simulink model "nn_12B_with_contracts_SLDV"  (R2019b)
settings: Solver=FixedStepDiscrete  StartTime=0  StopTime=100  FixedStep=1  RelTol=1e-3  EnableMultiTasking=on
model workspace (MAT data in the model file):
  ContractValidatorBlocksMap : containers.Map (value not decoded)
undefined symbols (not defined in the file): b1, b2, b3, meaninp, meanout, oostdinp, stdevout, w1, w2, w3, xinmax, xinmin
libraries: sldvlib x5, cocosimLibs x4
(part 2 of 2)

== system nn_12B_with_contracts_SLDV/nn_2x10x10x1/Neuron Layer 1/Neuron 3/If Action Subsystem1 ==
  In1 : Inport
  Action Port : ActionPort  ActionPortLabel=elseif(u1 < 0)
  Product1 : Product  RndMeth=Zero
  Sum3 : Sum  Inputs=|++
  bias4 : Constant  Value=2
  Out1 : Outport  VectorParamsAs1DForOutWhenUnconnected=off
  wires:
  In1/1 -> Product1/1, Sum3/1
  bias4/1 -> Sum3/2
  Sum3/1 -> Product1/2
  Product1/1 -> Out1/1

== system nn_12B_with_contracts_SLDV/nn_2x10x10x1/Neuron Layer 1/Neuron 3/If Action Subsystem2 ==
  In1 : Inport
  Action Port : ActionPort  ActionPortLabel=elseif( u1<0.995)
  Product1 : Product  RndMeth=Zero
  Sum3 : Sum  Inputs=|-+
  bias4 : Constant  Value=2
  Out1 : Outport  VectorParamsAs1DForOutWhenUnconnected=off
  wires:
  Product1/1 -> Out1/1
  Sum3/1 -> Product1/2
  bias4/1 -> Sum3/2
  In1/1 -> Sum3/1, Product1/1

== system nn_12B_with_contracts_SLDV/nn_2x10x10x1/Neuron Layer 1/Neuron 3/If Action Subsystem3 ==
  In1 : Inport
  Action Port : ActionPort  ActionPortLabel=else
  Sum : Sum  Inputs=|++
  bias1 : Constant  Value=0.990025
  weight1 : Gain  Gain=0.01
  Out1 : Outport  VectorParamsAs1DForOutWhenUnconnected=off
  wires:
  bias1/1 -> Sum/2
  weight1/1 -> Sum/1
  In1/1 -> weight1/1
  Sum/1 -> Out1/1

== system nn_12B_with_contracts_SLDV/nn_2x10x10x1/Neuron Layer 1/Neuron 4/If Action Subsystem ==
  In1 : Inport
  Action Port : ActionPort  ActionPortLabel=if(u1 < -0.995)
  Sum : Sum  Inputs=|+-
  bias1 : Constant  Value=0.990025
  weight1 : Gain  Gain=0.01
  Out1 : Outport  VectorParamsAs1DForOutWhenUnconnected=off
  wires:
  bias1/1 -> Sum/2
  weight1/1 -> Sum/1
  In1/1 -> weight1/1
  Sum/1 -> Out1/1

== system nn_12B_with_contracts_SLDV/nn_2x10x10x1/Neuron Layer 1/Neuron 4/If Action Subsystem1 ==
  In1 : Inport
  Action Port : ActionPort  ActionPortLabel=elseif(u1 < 0)
  Product1 : Product  RndMeth=Zero
  Sum3 : Sum  Inputs=|++
  bias4 : Constant  Value=2
  Out1 : Outport  VectorParamsAs1DForOutWhenUnconnected=off
  wires:
  In1/1 -> Product1/1, Sum3/1
  bias4/1 -> Sum3/2
  Sum3/1 -> Product1/2
  Product1/1 -> Out1/1

== system nn_12B_with_contracts_SLDV/nn_2x10x10x1/Neuron Layer 1/Neuron 4/If Action Subsystem2 ==
  In1 : Inport
  Action Port : ActionPort  ActionPortLabel=elseif( u1<0.995)
  Product1 : Product  RndMeth=Zero
  Sum3 : Sum  Inputs=|-+
  bias4 : Constant  Value=2
  Out1 : Outport  VectorParamsAs1DForOutWhenUnconnected=off
  wires:
  Product1/1 -> Out1/1
  Sum3/1 -> Product1/2
  bias4/1 -> Sum3/2
  In1/1 -> Sum3/1, Product1/1

== system nn_12B_with_contracts_SLDV/nn_2x10x10x1/Neuron Layer 1/Neuron 4/If Action Subsystem3 ==
  In1 : Inport
  Action Port : ActionPort  ActionPortLabel=else
  Sum : Sum  Inputs=|++
  bias1 : Constant  Value=0.990025
  weight1 : Gain  Gain=0.01
  Out1 : Outport  VectorParamsAs1DForOutWhenUnconnected=off
  wires:
  bias1/1 -> Sum/2
  weight1/1 -> Sum/1
  In1/1 -> weight1/1
  Sum/1 -> Out1/1

== system nn_12B_with_contracts_SLDV/nn_2x10x10x1/Neuron Layer 1/Neuron 5/If Action Subsystem ==
  In1 : Inport
  Action Port : ActionPort  ActionPortLabel=if(u1 < -0.995)
  Sum : Sum  Inputs=|+-
  bias1 : Constant  Value=0.990025
  weight1 : Gain  Gain=0.01
  Out1 : Outport  VectorParamsAs1DForOutWhenUnconnected=off
  wires:
  bias1/1 -> Sum/2
  weight1/1 -> Sum/1
  In1/1 -> weight1/1
  Sum/1 -> Out1/1

== system nn_12B_with_contracts_SLDV/nn_2x10x10x1/Neuron Layer 1/Neuron 5/If Action Subsystem1 ==
  In1 : Inport
  Action Port : ActionPort  ActionPortLabel=elseif(u1 < 0)
  Product1 : Product  RndMeth=Zero
  Sum3 : Sum  Inputs=|++
  bias4 : Constant  Value=2
  Out1 : Outport  VectorParamsAs1DForOutWhenUnconnected=off
  wires:
  In1/1 -> Product1/1, Sum3/1
  bias4/1 -> Sum3/2
  Sum3/1 -> Product1/2
  Product1/1 -> Out1/1

== system nn_12B_with_contracts_SLDV/nn_2x10x10x1/Neuron Layer 1/Neuron 5/If Action Subsystem2 ==
  In1 : Inport
  Action Port : ActionPort  ActionPortLabel=elseif( u1<0.995)
  Product1 : Product  RndMeth=Zero
  Sum3 : Sum  Inputs=|-+
  bias4 : Constant  Value=2
  Out1 : Outport  VectorParamsAs1DForOutWhenUnconnected=off
  wires:
  Product1/1 -> Out1/1
  Sum3/1 -> Product1/2
  bias4/1 -> Sum3/2
  In1/1 -> Sum3/1, Product1/1

== system nn_12B_with_contracts_SLDV/nn_2x10x10x1/Neuron Layer 1/Neuron 5/If Action Subsystem3 ==
  In1 : Inport
  Action Port : ActionPort  ActionPortLabel=else
  Sum : Sum  Inputs=|++
  bias1 : Constant  Value=0.990025
  weight1 : Gain  Gain=0.01
  Out1 : Outport  VectorParamsAs1DForOutWhenUnconnected=off
  wires:
  bias1/1 -> Sum/2
  weight1/1 -> Sum/1
  In1/1 -> weight1/1
  Sum/1 -> Out1/1

== system nn_12B_with_contracts_SLDV/nn_2x10x10x1/Neuron Layer 1/Neuron 6/If Action Subsystem ==
  In1 : Inport
  Action Port : ActionPort  ActionPortLabel=if(u1 < -0.995)
  Sum : Sum  Inputs=|+-
  bias1 : Constant  Value=0.990025
  weight1 : Gain  Gain=0.01
  Out1 : Outport  VectorParamsAs1DForOutWhenUnconnected=off
  wires:
  Sum/1 -> Out1/1
  In1/1 -> weight1/1
  weight1/1 -> Sum/1
  bias1/1 -> Sum/2

== system nn_12B_with_contracts_SLDV/nn_2x10x10x1/Neuron Layer 1/Neuron 6/If Action Subsystem1 ==
  In1 : Inport
  Action Port : ActionPort  ActionPortLabel=elseif(u1 < 0)
  Product1 : Product  RndMeth=Zero
  Sum3 : Sum  Inputs=|++
  bias4 : Constant  Value=2
  Out1 : Outport  VectorParamsAs1DForOutWhenUnconnected=off
  wires:
  Product1/1 -> Out1/1
  Sum3/1 -> Product1/2
  bias4/1 -> Sum3/2
  In1/1 -> Sum3/1, Product1/1

== system nn_12B_with_contracts_SLDV/nn_2x10x10x1/Neuron Layer 1/Neuron 6/If Action Subsystem2 ==
  In1 : Inport
  Action Port : ActionPort  ActionPortLabel=elseif( u1<0.995)
  Product1 : Product  RndMeth=Zero
  Sum3 : Sum  Inputs=|-+
  bias4 : Constant  Value=2
  Out1 : Outport  VectorParamsAs1DForOutWhenUnconnected=off
  wires:
  In1/1 -> Product1/1, Sum3/1
  bias4/1 -> Sum3/2
  Sum3/1 -> Product1/2
  Product1/1 -> Out1/1

== system nn_12B_with_contracts_SLDV/nn_2x10x10x1/Neuron Layer 1/Neuron 6/If Action Subsystem3 ==
  In1 : Inport
  Action Port : ActionPort  ActionPortLabel=else
  Sum : Sum  Inputs=|++
  bias1 : Constant  Value=0.990025
  weight1 : Gain  Gain=0.01
  Out1 : Outport  VectorParamsAs1DForOutWhenUnconnected=off
  wires:
  Sum/1 -> Out1/1
  In1/1 -> weight1/1
  weight1/1 -> Sum/1
  bias1/1 -> Sum/2

== system nn_12B_with_contracts_SLDV/nn_2x10x10x1/Neuron Layer 1/Neuron 7/If Action Subsystem ==
  In1 : Inport
  Action Port : ActionPort  ActionPortLabel=if(u1 < -0.995)
  Sum : Sum  Inputs=|+-
  bias1 : Constant  Value=0.990025
  weight1 : Gain  Gain=0.01
  Out1 : Outport  VectorParamsAs1DForOutWhenUnconnected=off
  wires:
  bias1/1 -> Sum/2
  weight1/1 -> Sum/1
  In1/1 -> weight1/1
  Sum/1 -> Out1/1

== system nn_12B_with_contracts_SLDV/nn_2x10x10x1/Neuron Layer 1/Neuron 7/If Action Subsystem1 ==
  In1 : Inport
  Action Port : ActionPort  ActionPortLabel=elseif(u1 < 0)
  Product1 : Product  RndMeth=Zero
  Sum3 : Sum  Inputs=|++
  bias4 : Constant  Value=2
  Out1 : Outport  VectorParamsAs1DForOutWhenUnconnected=off
  wires:
  In1/1 -> Product1/1, Sum3/1
  bias4/1 -> Sum3/2
  Sum3/1 -> Product1/2
  Product1/1 -> Out1/1

== system nn_12B_with_contracts_SLDV/nn_2x10x10x1/Neuron Layer 1/Neuron 7/If Action Subsystem2 ==
  In1 : Inport
  Action Port : ActionPort  ActionPortLabel=elseif( u1<0.995)
  Product1 : Product  RndMeth=Zero
  Sum3 : Sum  Inputs=|-+
  bias4 : Constant  Value=2
  Out1 : Outport  VectorParamsAs1DForOutWhenUnconnected=off
  wires:
  Product1/1 -> Out1/1
  Sum3/1 -> Product1/2
  bias4/1 -> Sum3/2
  In1/1 -> Sum3/1, Product1/1

== system nn_12B_with_contracts_SLDV/nn_2x10x10x1/Neuron Layer 1/Neuron 7/If Action Subsystem3 ==
  In1 : Inport
  Action Port : ActionPort  ActionPortLabel=else
  Sum : Sum  Inputs=|++
  bias1 : Constant  Value=0.990025
  weight1 : Gain  Gain=0.01
  Out1 : Outport  VectorParamsAs1DForOutWhenUnconnected=off
  wires:
  bias1/1 -> Sum/2
  weight1/1 -> Sum/1
  In1/1 -> weight1/1
  Sum/1 -> Out1/1

== system nn_12B_with_contracts_SLDV/nn_2x10x10x1/Neuron Layer 1/Neuron 8/If Action Subsystem ==
  In1 : Inport
  Action Port : ActionPort  ActionPortLabel=if(u1 < -0.995)
  Sum : Sum  Inputs=|+-
  bias1 : Constant  Value=0.990025
  weight1 : Gain  Gain=0.01
  Out1 : Outport  VectorParamsAs1DForOutWhenUnconnected=off
  wires:
  bias1/1 -> Sum/2
  weight1/1 -> Sum/1
  In1/1 -> weight1/1
  Sum/1 -> Out1/1

== system nn_12B_with_contracts_SLDV/nn_2x10x10x1/Neuron Layer 1/Neuron 8/If Action Subsystem1 ==
  In1 : Inport
  Action Port : ActionPort  ActionPortLabel=elseif(u1 < 0)
  Product1 : Product  RndMeth=Zero
  Sum3 : Sum  Inputs=|++
  bias4 : Constant  Value=2
  Out1 : Outport  VectorParamsAs1DForOutWhenUnconnected=off
  wires:
  In1/1 -> Product1/1, Sum3/1
  bias4/1 -> Sum3/2
  Sum3/1 -> Product1/2
  Product1/1 -> Out1/1

== system nn_12B_with_contracts_SLDV/nn_2x10x10x1/Neuron Layer 1/Neuron 8/If Action Subsystem2 ==
  In1 : Inport
  Action Port : ActionPort  ActionPortLabel=elseif( u1<0.995)
  Product1 : Product  RndMeth=Zero
  Sum3 : Sum  Inputs=|-+
  bias4 : Constant  Value=2
  Out1 : Outport  VectorParamsAs1DForOutWhenUnconnected=off
  wires:
  Product1/1 -> Out1/1
  Sum3/1 -> Product1/2
  bias4/1 -> Sum3/2
  In1/1 -> Sum3/1, Product1/1

== system nn_12B_with_contracts_SLDV/nn_2x10x10x1/Neuron Layer 1/Neuron 8/If Action Subsystem3 ==
  In1 : Inport
  Action Port : ActionPort  ActionPortLabel=else
  Sum : Sum  Inputs=|++
  bias1 : Constant  Value=0.990025
  weight1 : Gain  Gain=0.01
  Out1 : Outport  VectorParamsAs1DForOutWhenUnconnected=off
  wires:
  bias1/1 -> Sum/2
  weight1/1 -> Sum/1
  In1/1 -> weight1/1
  Sum/1 -> Out1/1

== system nn_12B_with_contracts_SLDV/nn_2x10x10x1/Neuron Layer 1/Neuron 9/If Action Subsystem ==
  In1 : Inport
  Action Port : ActionPort  ActionPortLabel=if(u1 < -0.995)
  Sum : Sum  Inputs=|+-
  bias1 : Constant  Value=0.990025
  weight1 : Gain  Gain=0.01
  Out1 : Outport  VectorParamsAs1DForOutWhenUnconnected=off
  wires:
  bias1/1 -> Sum/2
  weight1/1 -> Sum/1
  In1/1 -> weight1/1
  Sum/1 -> Out1/1

== system nn_12B_with_contracts_SLDV/nn_2x10x10x1/Neuron Layer 1/Neuron 9/If Action Subsystem1 ==
  In1 : Inport
  Action Port : ActionPort  ActionPortLabel=elseif(u1 < 0)
  Product1 : Product  RndMeth=Zero
  Sum3 : Sum  Inputs=|++
  bias4 : Constant  Value=2
  Out1 : Outport  VectorParamsAs1DForOutWhenUnconnected=off
  wires:
  In1/1 -> Product1/1, Sum3/1
  bias4/1 -> Sum3/2
  Sum3/1 -> Product1/2
  Product1/1 -> Out1/1

== system nn_12B_with_contracts_SLDV/nn_2x10x10x1/Neuron Layer 1/Neuron 9/If Action Subsystem2 ==
  In1 : Inport
  Action Port : ActionPort  ActionPortLabel=elseif( u1<0.995)
  Product1 : Product  RndMeth=Zero
  Sum3 : Sum  Inputs=|-+
  bias4 : Constant  Value=2
  Out1 : Outport  VectorParamsAs1DForOutWhenUnconnected=off
  wires:
  Product1/1 -> Out1/1
  Sum3/1 -> Product1/2
  bias4/1 -> Sum3/2
  In1/1 -> Sum3/1, Product1/1

== system nn_12B_with_contracts_SLDV/nn_2x10x10x1/Neuron Layer 1/Neuron 9/If Action Subsystem3 ==
  In1 : Inport
  Action Port : ActionPort  ActionPortLabel=else
  Sum : Sum  Inputs=|++
  bias1 : Constant  Value=0.990025
  weight1 : Gain  Gain=0.01
  Out1 : Outport  VectorParamsAs1DForOutWhenUnconnected=off
  wires:
  bias1/1 -> Sum/2
  weight1/1 -> Sum/1
  In1/1 -> weight1/1
  Sum/1 -> Out1/1

== system nn_12B_with_contracts_SLDV/nn_2x10x10x1/Neuron Layer 2/Neuron 1/If Action Subsystem ==
  In1 : Inport
  Action Port : ActionPort  ActionPortLabel=if(u1 < -0.995)
  Sum : Sum  Inputs=|+-
  bias1 : Constant  Value=0.990025
  weight1 : Gain  Gain=0.01
  Out1 : Outport  VectorParamsAs1DForOutWhenUnconnected=off
  wires:
  bias1/1 -> Sum/2
  weight1/1 -> Sum/1
  In1/1 -> weight1/1
  Sum/1 -> Out1/1

== system nn_12B_with_contracts_SLDV/nn_2x10x10x1/Neuron Layer 2/Neuron 1/If Action Subsystem1 ==
  In1 : Inport
  Action Port : ActionPort  ActionPortLabel=elseif(u1 < 0)
  Product1 : Product  RndMeth=Zero
  Sum3 : Sum  Inputs=|++
  bias4 : Constant  Value=2
  Out1 : Outport  VectorParamsAs1DForOutWhenUnconnected=off
  wires:
  In1/1 -> Product1/1, Sum3/1
  bias4/1 -> Sum3/2
  Sum3/1 -> Product1/2
  Product1/1 -> Out1/1

== system nn_12B_with_contracts_SLDV/nn_2x10x10x1/Neuron Layer 2/Neuron 1/If Action Subsystem2 ==
  In1 : Inport
  Action Port : ActionPort  ActionPortLabel=elseif( u1<0.995)
  Product1 : Product  RndMeth=Zero
  Sum3 : Sum  Inputs=|-+
  bias4 : Constant  Value=2
  Out1 : Outport  VectorParamsAs1DForOutWhenUnconnected=off
  wires:
  Product1/1 -> Out1/1
  Sum3/1 -> Product1/2
  bias4/1 -> Sum3/2
  In1/1 -> Sum3/1, Product1/1

== system nn_12B_with_contracts_SLDV/nn_2x10x10x1/Neuron Layer 2/Neuron 1/If Action Subsystem3 ==
  In1 : Inport
  Action Port : ActionPort  ActionPortLabel=else
  Sum : Sum  Inputs=|++
  bias1 : Constant  Value=0.990025
  weight1 : Gain  Gain=0.01
  Out1 : Outport  VectorParamsAs1DForOutWhenUnconnected=off
  wires:
  bias1/1 -> Sum/2
  weight1/1 -> Sum/1
  In1/1 -> weight1/1
  Sum/1 -> Out1/1

== system nn_12B_with_contracts_SLDV/nn_2x10x10x1/Neuron Layer 2/Neuron 10/If Action Subsystem ==
  In1 : Inport
  Action Port : ActionPort  ActionPortLabel=if(u1 < -0.995)
  Sum : Sum  Inputs=|+-
  bias1 : Constant  Value=0.990025
  weight1 : Gain  Gain=0.01
  Out1 : Outport  VectorParamsAs1DForOutWhenUnconnected=off
  wires:
  Sum/1 -> Out1/1
  In1/1 -> weight1/1
  weight1/1 -> Sum/1
  bias1/1 -> Sum/2

== system nn_12B_with_contracts_SLDV/nn_2x10x10x1/Neuron Layer 2/Neuron 10/If Action Subsystem1 ==
  In1 : Inport
  Action Port : ActionPort  ActionPortLabel=elseif(u1 < 0)
  Product1 : Product  RndMeth=Zero
  Sum3 : Sum  Inputs=|++
  bias4 : Constant  Value=2
  Out1 : Outport  VectorParamsAs1DForOutWhenUnconnected=off
  wires:
  Product1/1 -> Out1/1
  Sum3/1 -> Product1/2
  bias4/1 -> Sum3/2
  In1/1 -> Sum3/1, Product1/1

== system nn_12B_with_contracts_SLDV/nn_2x10x10x1/Neuron Layer 2/Neuron 10/If Action Subsystem2 ==
  In1 : Inport
  Action Port : ActionPort  ActionPortLabel=elseif( u1<0.995)
  Product1 : Product  RndMeth=Zero
  Sum3 : Sum  Inputs=|-+
  bias4 : Constant  Value=2
  Out1 : Outport  VectorParamsAs1DForOutWhenUnconnected=off
  wires:
  In1/1 -> Product1/1, Sum3/1
  bias4/1 -> Sum3/2
  Sum3/1 -> Product1/2
  Product1/1 -> Out1/1

== system nn_12B_with_contracts_SLDV/nn_2x10x10x1/Neuron Layer 2/Neuron 10/If Action Subsystem3 ==
  In1 : Inport
  Action Port : ActionPort  ActionPortLabel=else
  Sum : Sum  Inputs=|++
  bias1 : Constant  Value=0.990025
  weight1 : Gain  Gain=0.01
  Out1 : Outport  VectorParamsAs1DForOutWhenUnconnected=off
  wires:
  Sum/1 -> Out1/1
  In1/1 -> weight1/1
  weight1/1 -> Sum/1
  bias1/1 -> Sum/2

== system nn_12B_with_contracts_SLDV/nn_2x10x10x1/Neuron Layer 2/Neuron 2/If Action Subsystem ==
  In1 : Inport
  Action Port : ActionPort  ActionPortLabel=if(u1 < -0.995)
  Sum : Sum  Inputs=|+-
  bias1 : Constant  Value=0.990025
  weight1 : Gain  Gain=0.01
  Out1 : Outport  VectorParamsAs1DForOutWhenUnconnected=off
  wires:
  Sum/1 -> Out1/1
  In1/1 -> weight1/1
  weight1/1 -> Sum/1
  bias1/1 -> Sum/2

== system nn_12B_with_contracts_SLDV/nn_2x10x10x1/Neuron Layer 2/Neuron 2/If Action Subsystem1 ==
  In1 : Inport
  Action Port : ActionPort  ActionPortLabel=elseif(u1 < 0)
  Product1 : Product  RndMeth=Zero
  Sum3 : Sum  Inputs=|++
  bias4 : Constant  Value=2
  Out1 : Outport  VectorParamsAs1DForOutWhenUnconnected=off
  wires:
  Product1/1 -> Out1/1
  Sum3/1 -> Product1/2
  bias4/1 -> Sum3/2
  In1/1 -> Sum3/1, Product1/1

== system nn_12B_with_contracts_SLDV/nn_2x10x10x1/Neuron Layer 2/Neuron 2/If Action Subsystem2 ==
  In1 : Inport
  Action Port : ActionPort  ActionPortLabel=elseif( u1<0.995)
  Product1 : Product  RndMeth=Zero
  Sum3 : Sum  Inputs=|-+
  bias4 : Constant  Value=2
  Out1 : Outport  VectorParamsAs1DForOutWhenUnconnected=off
  wires:
  In1/1 -> Product1/1, Sum3/1
  bias4/1 -> Sum3/2
  Sum3/1 -> Product1/2
  Product1/1 -> Out1/1

== system nn_12B_with_contracts_SLDV/nn_2x10x10x1/Neuron Layer 2/Neuron 2/If Action Subsystem3 ==
  In1 : Inport
  Action Port : ActionPort  ActionPortLabel=else
  Sum : Sum  Inputs=|++
  bias1 : Constant  Value=0.990025
  weight1 : Gain  Gain=0.01
  Out1 : Outport  VectorParamsAs1DForOutWhenUnconnected=off
  wires:
  Sum/1 -> Out1/1
  In1/1 -> weight1/1
  weight1/1 -> Sum/1
  bias1/1 -> Sum/2

== system nn_12B_with_contracts_SLDV/nn_2x10x10x1/Neuron Layer 2/Neuron 3/If Action Subsystem ==
  In1 : Inport
  Action Port : ActionPort  ActionPortLabel=if(u1 < -0.995)
  Sum : Sum  Inputs=|+-
  bias1 : Constant  Value=0.990025
  weight1 : Gain  Gain=0.01
  Out1 : Outport  VectorParamsAs1DForOutWhenUnconnected=off
  wires:
  bias1/1 -> Sum/2
  weight1/1 -> Sum/1
  In1/1 -> weight1/1
  Sum/1 -> Out1/1

== system nn_12B_with_contracts_SLDV/nn_2x10x10x1/Neuron Layer 2/Neuron 3/If Action Subsystem1 ==
  In1 : Inport
  Action Port : ActionPort  ActionPortLabel=elseif(u1 < 0)
  Product1 : Product  RndMeth=Zero
  Sum3 : Sum  Inputs=|++
  bias4 : Constant  Value=2
  Out1 : Outport  VectorParamsAs1DForOutWhenUnconnected=off
  wires:
  In1/1 -> Product1/1, Sum3/1
  bias4/1 -> Sum3/2
  Sum3/1 -> Product1/2
  Product1/1 -> Out1/1

== system nn_12B_with_contracts_SLDV/nn_2x10x10x1/Neuron Layer 2/Neuron 3/If Action Subsystem2 ==
  In1 : Inport
  Action Port : ActionPort  ActionPortLabel=elseif( u1<0.995)
  Product1 : Product  RndMeth=Zero
  Sum3 : Sum  Inputs=|-+
  bias4 : Constant  Value=2
  Out1 : Outport  VectorParamsAs1DForOutWhenUnconnected=off
  wires:
  Product1/1 -> Out1/1
  Sum3/1 -> Product1/2
  bias4/1 -> Sum3/2
  In1/1 -> Sum3/1, Product1/1

== system nn_12B_with_contracts_SLDV/nn_2x10x10x1/Neuron Layer 2/Neuron 3/If Action Subsystem3 ==
  In1 : Inport
  Action Port : ActionPort  ActionPortLabel=else
  Sum : Sum  Inputs=|++
  bias1 : Constant  Value=0.990025
  weight1 : Gain  Gain=0.01
  Out1 : Outport  VectorParamsAs1DForOutWhenUnconnected=off
  wires:
  bias1/1 -> Sum/2
  weight1/1 -> Sum/1
  In1/1 -> weight1/1
  Sum/1 -> Out1/1

== system nn_12B_with_contracts_SLDV/nn_2x10x10x1/Neuron Layer 2/Neuron 4/If Action Subsystem ==
  In1 : Inport
  Action Port : ActionPort  ActionPortLabel=if(u1 < -0.995)
  Sum : Sum  Inputs=|+-
  bias1 : Constant  Value=0.990025
  weight1 : Gain  Gain=0.01
  Out1 : Outport  VectorParamsAs1DForOutWhenUnconnected=off
  wires:
  bias1/1 -> Sum/2
  weight1/1 -> Sum/1
  In1/1 -> weight1/1
  Sum/1 -> Out1/1

== system nn_12B_with_contracts_SLDV/nn_2x10x10x1/Neuron Layer 2/Neuron 4/If Action Subsystem1 ==
  In1 : Inport
  Action Port : ActionPort  ActionPortLabel=elseif(u1 < 0)
  Product1 : Product  RndMeth=Zero
  Sum3 : Sum  Inputs=|++
  bias4 : Constant  Value=2
  Out1 : Outport  VectorParamsAs1DForOutWhenUnconnected=off
  wires:
  In1/1 -> Product1/1, Sum3/1
  bias4/1 -> Sum3/2
  Sum3/1 -> Product1/2
  Product1/1 -> Out1/1

== system nn_12B_with_contracts_SLDV/nn_2x10x10x1/Neuron Layer 2/Neuron 4/If Action Subsystem2 ==
  In1 : Inport
  Action Port : ActionPort  ActionPortLabel=elseif( u1<0.995)
  Product1 : Product  RndMeth=Zero
  Sum3 : Sum  Inputs=|-+
  bias4 : Constant  Value=2
  Out1 : Outport  VectorParamsAs1DForOutWhenUnconnected=off
  wires:
  Product1/1 -> Out1/1
  Sum3/1 -> Product1/2
  bias4/1 -> Sum3/2
  In1/1 -> Sum3/1, Product1/1

== system nn_12B_with_contracts_SLDV/nn_2x10x10x1/Neuron Layer 2/Neuron 4/If Action Subsystem3 ==
  In1 : Inport
  Action Port : ActionPort  ActionPortLabel=else
  Sum : Sum  Inputs=|++
  bias1 : Constant  Value=0.990025
  weight1 : Gain  Gain=0.01
  Out1 : Outport  VectorParamsAs1DForOutWhenUnconnected=off
  wires:
  bias1/1 -> Sum/2
  weight1/1 -> Sum/1
  In1/1 -> weight1/1
  Sum/1 -> Out1/1

== system nn_12B_with_contracts_SLDV/nn_2x10x10x1/Neuron Layer 2/Neuron 5/If Action Subsystem ==
  In1 : Inport
  Action Port : ActionPort  ActionPortLabel=if(u1 < -0.995)
  Sum : Sum  Inputs=|+-
  bias1 : Constant  Value=0.990025
  weight1 : Gain  Gain=0.01
  Out1 : Outport  VectorParamsAs1DForOutWhenUnconnected=off
  wires:
  bias1/1 -> Sum/2
  weight1/1 -> Sum/1
  In1/1 -> weight1/1
  Sum/1 -> Out1/1

== system nn_12B_with_contracts_SLDV/nn_2x10x10x1/Neuron Layer 2/Neuron 5/If Action Subsystem1 ==
  In1 : Inport
  Action Port : ActionPort  ActionPortLabel=elseif(u1 < 0)
  Product1 : Product  RndMeth=Zero
  Sum3 : Sum  Inputs=|++
  bias4 : Constant  Value=2
  Out1 : Outport  VectorParamsAs1DForOutWhenUnconnected=off
  wires:
  In1/1 -> Product1/1, Sum3/1
  bias4/1 -> Sum3/2
  Sum3/1 -> Product1/2
  Product1/1 -> Out1/1

== system nn_12B_with_contracts_SLDV/nn_2x10x10x1/Neuron Layer 2/Neuron 5/If Action Subsystem2 ==
  In1 : Inport
  Action Port : ActionPort  ActionPortLabel=elseif( u1<0.995)
  Product1 : Product  RndMeth=Zero
  Sum3 : Sum  Inputs=|-+
  bias4 : Constant  Value=2
  Out1 : Outport  VectorParamsAs1DForOutWhenUnconnected=off
  wires:
  Product1/1 -> Out1/1
  Sum3/1 -> Product1/2
  bias4/1 -> Sum3/2
  In1/1 -> Sum3/1, Product1/1

== system nn_12B_with_contracts_SLDV/nn_2x10x10x1/Neuron Layer 2/Neuron 5/If Action Subsystem3 ==
  In1 : Inport
  Action Port : ActionPort  ActionPortLabel=else
  Sum : Sum  Inputs=|++
  bias1 : Constant  Value=0.990025
  weight1 : Gain  Gain=0.01
  Out1 : Outport  VectorParamsAs1DForOutWhenUnconnected=off
  wires:
  bias1/1 -> Sum/2
  weight1/1 -> Sum/1
  In1/1 -> weight1/1
  Sum/1 -> Out1/1

== system nn_12B_with_contracts_SLDV/nn_2x10x10x1/Neuron Layer 2/Neuron 6/If Action Subsystem ==
  In1 : Inport
  Action Port : ActionPort  ActionPortLabel=if(u1 < -0.995)
  Sum : Sum  Inputs=|+-
  bias1 : Constant  Value=0.990025
  weight1 : Gain  Gain=0.01
  Out1 : Outport  VectorParamsAs1DForOutWhenUnconnected=off
  wires:
  Sum/1 -> Out1/1
  In1/1 -> weight1/1
  weight1/1 -> Sum/1
  bias1/1 -> Sum/2

== system nn_12B_with_contracts_SLDV/nn_2x10x10x1/Neuron Layer 2/Neuron 6/If Action Subsystem1 ==
  In1 : Inport
  Action Port : ActionPort  ActionPortLabel=elseif(u1 < 0)
  Product1 : Product  RndMeth=Zero
  Sum3 : Sum  Inputs=|++
  bias4 : Constant  Value=2
  Out1 : Outport  VectorParamsAs1DForOutWhenUnconnected=off
  wires:
  Product1/1 -> Out1/1
  Sum3/1 -> Product1/2
  bias4/1 -> Sum3/2
  In1/1 -> Sum3/1, Product1/1

== system nn_12B_with_contracts_SLDV/nn_2x10x10x1/Neuron Layer 2/Neuron 6/If Action Subsystem2 ==
  In1 : Inport
  Action Port : ActionPort  ActionPortLabel=elseif( u1<0.995)
  Product1 : Product  RndMeth=Zero
  Sum3 : Sum  Inputs=|-+
  bias4 : Constant  Value=2
  Out1 : Outport  VectorParamsAs1DForOutWhenUnconnected=off
  wires:
  In1/1 -> Product1/1, Sum3/1
  bias4/1 -> Sum3/2
  Sum3/1 -> Product1/2
  Product1/1 -> Out1/1

== system nn_12B_with_contracts_SLDV/nn_2x10x10x1/Neuron Layer 2/Neuron 6/If Action Subsystem3 ==
  In1 : Inport
  Action Port : ActionPort  ActionPortLabel=else
  Sum : Sum  Inputs=|++
  bias1 : Constant  Value=0.990025
  weight1 : Gain  Gain=0.01
  Out1 : Outport  VectorParamsAs1DForOutWhenUnconnected=off
  wires:
  Sum/1 -> Out1/1
  In1/1 -> weight1/1
  weight1/1 -> Sum/1
  bias1/1 -> Sum/2

== system nn_12B_with_contracts_SLDV/nn_2x10x10x1/Neuron Layer 2/Neuron 7/If Action Subsystem ==
  In1 : Inport
  Action Port : ActionPort  ActionPortLabel=if(u1 < -0.995)
  Sum : Sum  Inputs=|+-
  bias1 : Constant  Value=0.990025
  weight1 : Gain  Gain=0.01
  Out1 : Outport  VectorParamsAs1DForOutWhenUnconnected=off
  wires:
  bias1/1 -> Sum/2
  weight1/1 -> Sum/1
  In1/1 -> weight1/1
  Sum/1 -> Out1/1

== system nn_12B_with_contracts_SLDV/nn_2x10x10x1/Neuron Layer 2/Neuron 7/If Action Subsystem1 ==
  In1 : Inport
  Action Port : ActionPort  ActionPortLabel=elseif(u1 < 0)
  Product1 : Product  RndMeth=Zero
  Sum3 : Sum  Inputs=|++
  bias4 : Constant  Value=2
  Out1 : Outport  VectorParamsAs1DForOutWhenUnconnected=off
  wires:
  In1/1 -> Product1/1, Sum3/1
  bias4/1 -> Sum3/2
  Sum3/1 -> Product1/2
  Product1/1 -> Out1/1

== system nn_12B_with_contracts_SLDV/nn_2x10x10x1/Neuron Layer 2/Neuron 7/If Action Subsystem2 ==
  In1 : Inport
  Action Port : ActionPort  ActionPortLabel=elseif( u1<0.995)
  Product1 : Product  RndMeth=Zero
  Sum3 : Sum  Inputs=|-+
  bias4 : Constant  Value=2
  Out1 : Outport  VectorParamsAs1DForOutWhenUnconnected=off
  wires:
  Product1/1 -> Out1/1
  Sum3/1 -> Product1/2
  bias4/1 -> Sum3/2
  In1/1 -> Sum3/1, Product1/1

== system nn_12B_with_contracts_SLDV/nn_2x10x10x1/Neuron Layer 2/Neuron 7/If Action Subsystem3 ==
  In1 : Inport
  Action Port : ActionPort  ActionPortLabel=else
  Sum : Sum  Inputs=|++
  bias1 : Constant  Value=0.990025
  weight1 : Gain  Gain=0.01
  Out1 : Outport  VectorParamsAs1DForOutWhenUnconnected=off
  wires:
  bias1/1 -> Sum/2
  weight1/1 -> Sum/1
  In1/1 -> weight1/1
  Sum/1 -> Out1/1

== system nn_12B_with_contracts_SLDV/nn_2x10x10x1/Neuron Layer 2/Neuron 8/If Action Subsystem ==
  In1 : Inport
  Action Port : ActionPort  ActionPortLabel=if(u1 < -0.995)
  Sum : Sum  Inputs=|+-
  bias1 : Constant  Value=0.990025
  weight1 : Gain  Gain=0.01
  Out1 : Outport  VectorParamsAs1DForOutWhenUnconnected=off
  wires:
  bias1/1 -> Sum/2
  weight1/1 -> Sum/1
  In1/1 -> weight1/1
  Sum/1 -> Out1/1

== system nn_12B_with_contracts_SLDV/nn_2x10x10x1/Neuron Layer 2/Neuron 8/If Action Subsystem1 ==
  In1 : Inport
  Action Port : ActionPort  ActionPortLabel=elseif(u1 < 0)
  Product1 : Product  RndMeth=Zero
  Sum3 : Sum  Inputs=|++
  bias4 : Constant  Value=2
  Out1 : Outport  VectorParamsAs1DForOutWhenUnconnected=off
  wires:
  In1/1 -> Product1/1, Sum3/1
  bias4/1 -> Sum3/2
  Sum3/1 -> Product1/2
  Product1/1 -> Out1/1

== system nn_12B_with_contracts_SLDV/nn_2x10x10x1/Neuron Layer 2/Neuron 8/If Action Subsystem2 ==
  In1 : Inport
  Action Port : ActionPort  ActionPortLabel=elseif( u1<0.995)
  Product1 : Product  RndMeth=Zero
  Sum3 : Sum  Inputs=|-+
  bias4 : Constant  Value=2
  Out1 : Outport  VectorParamsAs1DForOutWhenUnconnected=off
  wires:
  Product1/1 -> Out1/1
  Sum3/1 -> Product1/2
  bias4/1 -> Sum3/2
  In1/1 -> Sum3/1, Product1/1

== system nn_12B_with_contracts_SLDV/nn_2x10x10x1/Neuron Layer 2/Neuron 8/If Action Subsystem3 ==
  In1 : Inport
  Action Port : ActionPort  ActionPortLabel=else
  Sum : Sum  Inputs=|++
  bias1 : Constant  Value=0.990025
  weight1 : Gain  Gain=0.01
  Out1 : Outport  VectorParamsAs1DForOutWhenUnconnected=off
  wires:
  bias1/1 -> Sum/2
  weight1/1 -> Sum/1
  In1/1 -> weight1/1
  Sum/1 -> Out1/1

== system nn_12B_with_contracts_SLDV/nn_2x10x10x1/Neuron Layer 2/Neuron 9/If Action Subsystem ==
  In1 : Inport
  Action Port : ActionPort  ActionPortLabel=if(u1 < -0.995)
  Sum : Sum  Inputs=|+-
  bias1 : Constant  Value=0.990025
  weight1 : Gain  Gain=0.01
  Out1 : Outport  VectorParamsAs1DForOutWhenUnconnected=off
  wires:
  bias1/1 -> Sum/2
  weight1/1 -> Sum/1
  In1/1 -> weight1/1
  Sum/1 -> Out1/1

== system nn_12B_with_contracts_SLDV/nn_2x10x10x1/Neuron Layer 2/Neuron 9/If Action Subsystem1 ==
  In1 : Inport
  Action Port : ActionPort  ActionPortLabel=elseif(u1 < 0)
  Product1 : Product  RndMeth=Zero
  Sum3 : Sum  Inputs=|++
  bias4 : Constant  Value=2
  Out1 : Outport  VectorParamsAs1DForOutWhenUnconnected=off
  wires:
  In1/1 -> Product1/1, Sum3/1
  bias4/1 -> Sum3/2
  Sum3/1 -> Product1/2
  Product1/1 -> Out1/1

== system nn_12B_with_contracts_SLDV/nn_2x10x10x1/Neuron Layer 2/Neuron 9/If Action Subsystem2 ==
  In1 : Inport
  Action Port : ActionPort  ActionPortLabel=elseif( u1<0.995)
  Product1 : Product  RndMeth=Zero
  Sum3 : Sum  Inputs=|-+
  bias4 : Constant  Value=2
  Out1 : Outport  VectorParamsAs1DForOutWhenUnconnected=off
  wires:
  Product1/1 -> Out1/1
  Sum3/1 -> Product1/2
  bias4/1 -> Sum3/2
  In1/1 -> Sum3/1, Product1/1

== system nn_12B_with_contracts_SLDV/nn_2x10x10x1/Neuron Layer 2/Neuron 9/If Action Subsystem3 ==
  In1 : Inport
  Action Port : ActionPort  ActionPortLabel=else
  Sum : Sum  Inputs=|++
  bias1 : Constant  Value=0.990025
  weight1 : Gain  Gain=0.01
  Out1 : Outport  VectorParamsAs1DForOutWhenUnconnected=off
  wires:
  bias1/1 -> Sum/2
  weight1/1 -> Sum/1
  In1/1 -> weight1/1
  Sum/1 -> Out1/1
